simulink model "vj6simulink"  (R2020b)
settings: Solver=VariableStepAuto  StartTime=0.0  StopTime=T  RelTol=1e-3
values from neighbouring files (symbols this model uses):
  K = 100    [vj6.m]
  m = 1.5    [vj6.m]
  vu = 0.002    [vj6.m]
settings Model: Creator=dominik  LastModifiedBy=dominik

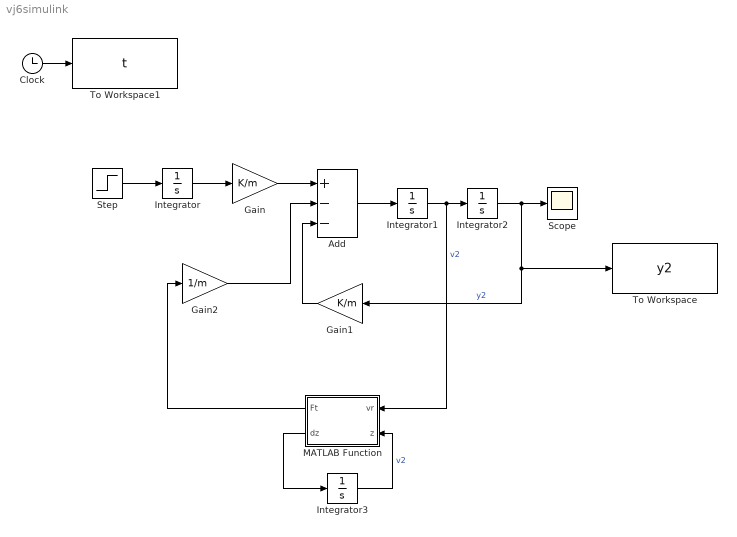
== system vj6simulink ==
  Add : Sum  Inputs=+--
  Clock : Clock
  Gain : Gain  Gain=K/m
  Gain1 : Gain  Gain=K/m
  Gain2 : Gain  Gain=1/m
  Integrator{,1..3} (4 alike) : Integrator
  MATLAB Function : MATLAB Function  TreatAsAtomicUnit=on
  Scope : Scope
  Step : Step  Time=0  After=vu  SampleTime=0
  To Workspace : ToWorkspace  VariableName=y2  SampleTime=-1
  To Workspace1 : ToWorkspace  VariableName=t  SampleTime=-1
  wires:
  Step/1 -> Integrator/1
  Integrator/1 -> Gain/1
  Gain/1 -> Add/1
  Add/1 -> Integrator1/1
  Integrator1/1 -> MATLAB Function/1(vr), Integrator2/1  "v2"
  Integrator2/1 -> To Workspace/1, Gain1/1, Scope/1  "y2"
  Gain1/1 -> Add/3
  MATLAB Function/2(dz) -> Integrator3/1
  Integrator3/1 -> MATLAB Function/2(z)  "v2"
  MATLAB Function/1(Ft) -> Gain2/1
  Gain2/1 -> Add/2
  Clock/1 -> To Workspace1/1

== matlab function vj6simulink/MATLAB Function ==
  data: vr input; Ft output; z input; dz output
function [Ft, dz] = trenje(vr, z)
a = 0.25;
sigma1 = 30;
sigma0 = 2e4;
z0 = 1e-5;

if (vr > 0 && z >= z0) || (vr < 0 && z <= -z0)
    dz = 0;
else
    dz = vr;
end

if abs(z) <= z0
    Ft = sigma0*(1 + a)*z + sigma1*dz;
else
    Ft = sigma0*z0*sign(z);
end


end
